simulink model "sample_R2018a"  (R2018a)
settings: Solver=ode4  StartTime=0.0  StopTime=5  FixedStep=0.001  RelTol=1e-3
settings Model: Creator=kawata  LastModifiedBy=kawata

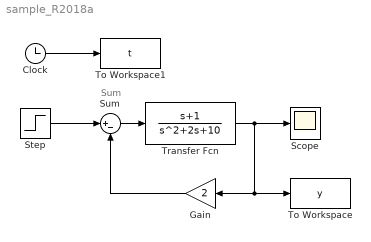
== system sample_R2018a ==
  note: Sum
  Clock : Clock
  Gain : Gain  Gain=2
  Scope : Scope
  Step : Step  SampleTime=0
  Sum : Sum  Inputs=|+-
  To Workspace : ToWorkspace  VariableName=y  SampleTime=-1
  To Workspace1 : ToWorkspace  VariableName=t  SampleTime=-1
  Transfer Fcn : TransferFcn  Numerator=[1 1]  Denominator=[1 2 10]
  wires:
  Clock/1 -> To Workspace1/1
  Sum/1 -> Transfer Fcn/1
  Transfer Fcn/1 -> Gain/1, To Workspace/1, Scope/1
  Gain/1 -> Sum/2
  Step/1 -> Sum/1
